simulink subsystem "SubSystemHubmagnet"  (R2020b)
settings: Solver=VariableStepAuto  StartTime=0.0  StopTime=10.0  RelTol=1e-3
settings Model: Creator=kaebi  LastModifiedBy=kaebi

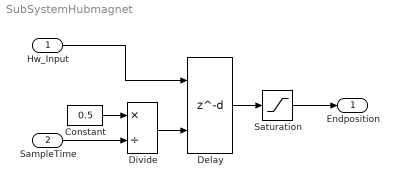
== system SubSystemHubmagnet ==
  Hw_Input : Inport
  SampleTime : Inport  Port=2
  Constant : Constant  Value=0.5
  Delay : Delay  DelayLengthSource=Input port  DelayLengthUpperLimit=2500
      settings: InputPortMap=u0,p1
  Divide : Product  Inputs=*/
  Saturation : Saturate  UpperLimit=1  LowerLimit=0
  Endposition : Outport
  wires:
  Saturation/1 -> Endposition/1
  Hw_Input/1 -> Delay/1
  Delay/1 -> Saturation/1
  Divide/1 -> Delay/2
  Constant/1 -> Divide/1
  SampleTime/1 -> Divide/2
